simulink model "Stanley02"  (R2023a)
settings: Solver=VariableStepAuto  StartTime=0.0  StopTime=120  RelTol=1e-3
values from neighbouring files (symbols this model uses):
  r_yaw = atan2(dif_yyyy , dif_xxxx)    [stanley_ref_final.m]
undefined symbols (not defined in the file or in its folder): cx, cy
libraries: Solver_SF x1, simulink x1
settings Model: Creator=ASUS  LastModifiedBy=ASUS

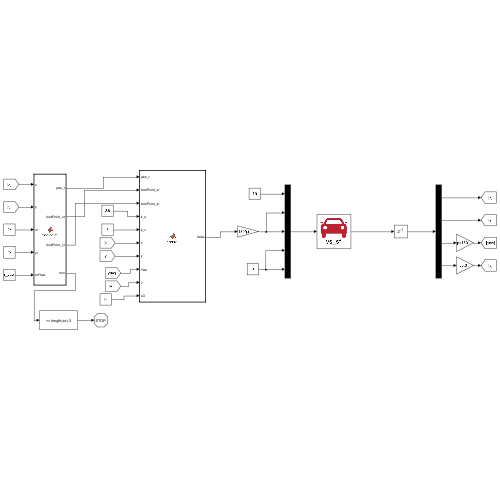
[thumbnail: Simulink's stored preview of the top-level diagram]
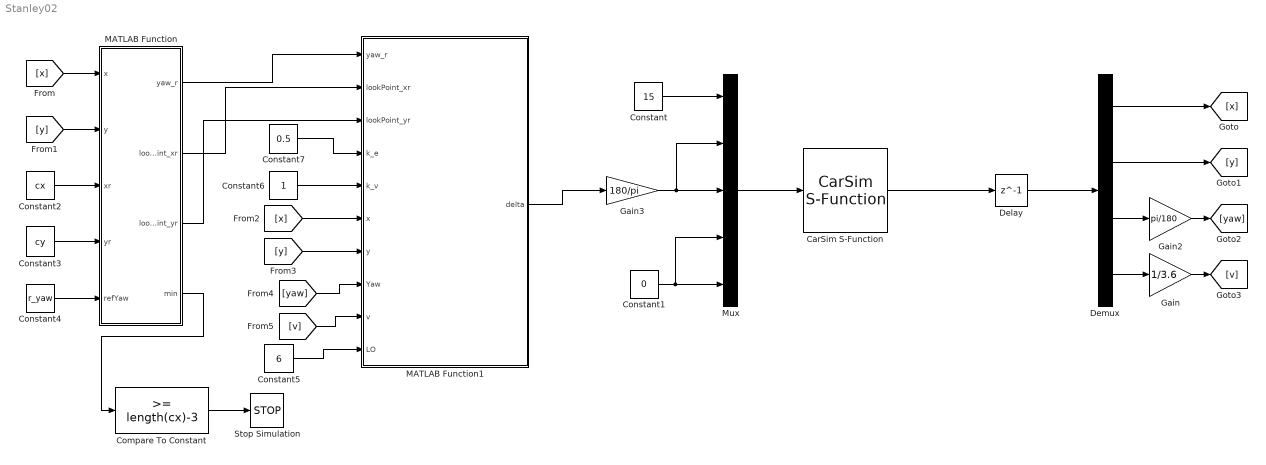
== system Stanley02 ==
  CarSim S-Function : Solver_SF/CarSim S-Function  Priority=1  SIMFILE=simfile.sim
  Compare To Constant : simulink/Logic and Bit Operations/Compare To Constant  relop=>=  const=length(cx)-3  OutDataTypeStr=boolean
  Constant : Constant  Value=15
  Constant1 : Constant  Value=0
  Constant2 : Constant  Value=cx
  Constant3 : Constant  Value=cy
  Constant4 : Constant  Value=r_yaw
  Constant5 : Constant  Value=6
  Constant6 : Constant
  Constant7 : Constant  Value=0.5
  Delay : Delay  DelayLength=1
  Demux : Demux
  Gain : Gain  Gain=1/3.6
  Gain2 : Gain  Gain=pi/180
  Gain3 : Gain  Gain=180/pi
  MATLAB Function : MATLAB Function  TreatAsAtomicUnit=on
  MATLAB Function1 : MATLAB Function  TreatAsAtomicUnit=on
  Mux : Mux  Inputs=5
  Stop Simulation : Stop
  wires:
  CarSim S-Function/1 -> Delay/1
  Demux/1 -> [x]
  Demux/2 -> [y]
  Demux/3 -> Gain2/1
  Demux/4 -> Gain/1
  Gain/1 -> [v]
  Gain2/1 -> [yaw]
  Delay/1 -> Demux/1
  Constant/1 -> Mux/1
  Gain3/1 -> Mux/2, Mux/3
  Constant1/1 -> Mux/4, Mux/5
  Mux/1 -> CarSim S-Function/1
  [x] -> MATLAB Function/1(x)
  [y] -> MATLAB Function/2(y)
  Constant2/1 -> MATLAB Function/3(xr)
  Constant3/1 -> MATLAB Function/4(yr)
  Constant4/1 -> MATLAB Function/5(refYaw)
  MATLAB Function/4(min) -> Compare To Constant/1
  Constant5/1 -> MATLAB Function1/10(LO)
  Constant6/1 -> MATLAB Function1/5(k_v)
  Constant7/1 -> MATLAB Function1/4(k_e)
  [y] -> MATLAB Function1/7(y)
  [x] -> MATLAB Function1/6(x)
  [yaw] -> MATLAB Function1/8(Yaw)
  [v] -> MATLAB Function1/9(v)
  MATLAB Function/1(yaw_r) -> MATLAB Function1/1(yaw_r)
  MATLAB Function/2(lookPoint_xr) -> MATLAB Function1/2(lookPoint_xr)
  MATLAB Function/3(lookPoint_yr) -> MATLAB Function1/3(lookPoint_yr)
  MATLAB Function1/1(delta) -> Gain3/1
  Compare To Constant/1 -> Stop Simulation/1

== matlab function Stanley02/MATLAB Function1 ==
  data: yaw_r input; delta output; lookPoint_xr input; lookPoint_yr input; k_e input; k_v input; x input; y input; Yaw input; v input; LO input
function delta = control(yaw_r,lookPoint_xr,lookPoint_yr,k_e,k_v,x,y,Yaw,v,LO)

e_y=sqrt((x-lookPoint_xr)^2+(y-lookPoint_yr)^2);

dx=x-lookPoint_xr;
dy=y-lookPoint_yr;
L_R = dy*cos(Yaw) - dx*sin(Yaw);

if L_R < 0
   e_y = -e_y;     
end

ey_yaw=atan2(-k_e*e_y,k_v*v+LO);

if ey_yaw > pi
    ey_yaw = ey_yaw - 2*pi;
end
if ey_yaw < -pi
    ey_yaw = ey_yaw + 2*pi;
end

ehead_yaw=yaw_r-Yaw;

if ehead_yaw > pi
    ehead_yaw = ehead_yaw - 2*pi;
end
if ehead_yaw < -pi
    ehead_yaw = ehead_yaw + 2*pi;
end


delta = ehead_yaw+ey_yaw;

if delta > pi/6
    delta = pi/6;
end
if delta < -pi/6
    delta = -pi/6;
end

end

== matlab function Stanley02/MATLAB Function ==
  data: x input; yaw_r output; y input; xr input; yr input; refYaw input; lookPoint_xr output; lookPoint_yr output; min output
function [yaw_r,lookPoint_xr, lookPoint_yr,min] = findPoint(x,y, xr,yr,refYaw)

n=length(xr);
d_min=(x-xr(1))^2+(y-yr(1))^2;
min=1;
for i = 1:n
    d = (x-xr(i))^2+(y-yr(i))^2; 
    if d<d_min
        d_min=d;
        min=i;
    end
end

lookPoint_xr = xr(min);
lookPoint_yr = yr(min);
yaw_r=refYaw(min);

end
